simulink model "Trajectory"  (R2025a)
settings: Solver=VariableStepAuto  StartTime=0.0  StopTime=30  FixedStep=0.01  RelTol=1e-3
values from neighbouring files (symbols this model uses):
  P = [     0   0 ... (first row only)    [untitled2.m]
  s = 5    [untitled2.m]
libraries: robotalgslib x1
settings Model: Creator=mwali  LastModifiedBy=mwali

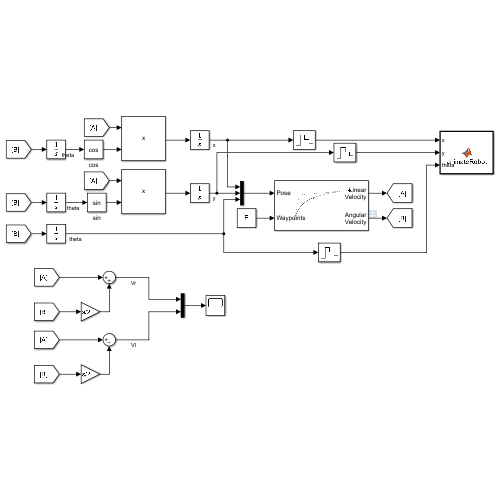
[thumbnail: Simulink's stored preview of the top-level diagram]
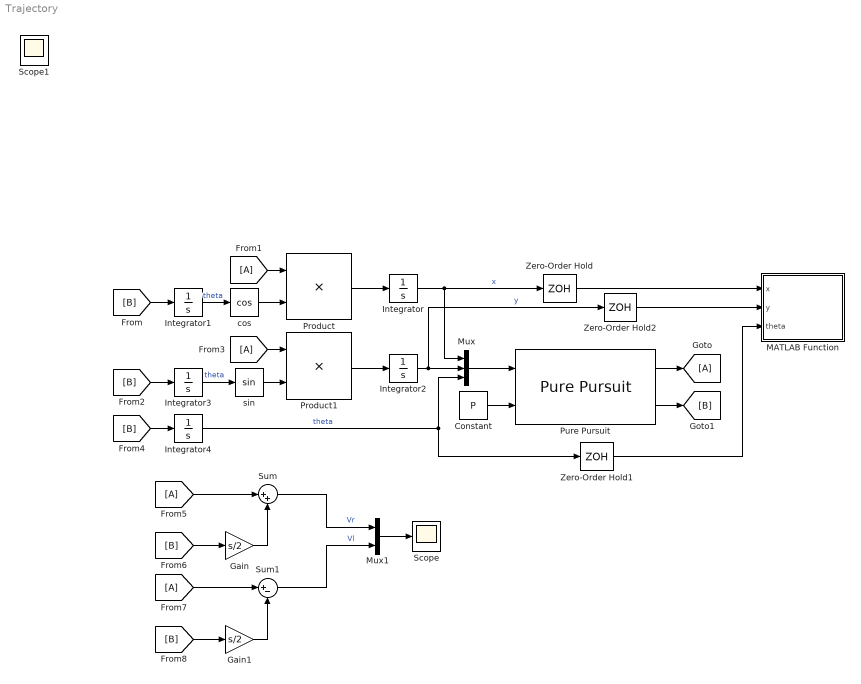
== system Trajectory ==
  Constant : Constant  Value=P
  From{1,3,5,7} (4 alike) : From
  Gain : Gain  Gain=s/2
  Gain1 : Gain  Gain=s/2
  Goto : Goto
  Integrator{,1..4} (5 alike) : Integrator
  MATLAB Function : MATLAB Function  TreatAsAtomicUnit=on
  Mux : Mux  Inputs=3
  Mux1 : Mux  Inputs=2
  Product : Product
  Product1 : Product
  Pure Pursuit : robotalgslib/Pure Pursuit  DesiredLinearVelocityPort=off  DesiredLinearVelocity=0.15  MaxAngularVelocity=1.0  LookaheadDistancePort=off  LookaheadDistance=1.2  TargetDirPort=off  SimulateUsing=Code generation
      settings: LibrarySourceBlock=robotmobilelib/Pure Pursuit
  Scope : Scope
      settings: ActiveDisplayYMinimum=-1.3727035211846959  ActiveDisplayYMaximum=2.3727035211846963
  Sum : Sum  Inputs=|++
  Sum1 : Sum  Inputs=|+-
  Zero-Order Hold : ZeroOrderHold  SampleTime=0.01
  Zero-Order Hold1 : ZeroOrderHold  SampleTime=0.01
  Zero-Order Hold2 : ZeroOrderHold  SampleTime=0.01
  cos : Trigonometry  Operator=cos
  sin : Trigonometry
  Scope1 : Scope
      settings: ActiveDisplayYMinimum=-1  ActiveDisplayYMaximum=1
  wires:
  Product/1 -> Integrator/1
  cos/1 -> Product/2
  Integrator1/1 -> cos/1  "theta"
  [B] -> Integrator1/1
  From1/1 -> Product/1
  Pure Pursuit/1 -> Goto/1
  Pure Pursuit/2 -> [B]
  Integrator/1 -> Zero-Order Hold/1, Mux/1  "x"
  sin/1 -> Product1/2
  Integrator2/1 -> Mux/2, Zero-Order Hold2/1  "y"
  [B] -> Integrator3/1
  Product1/1 -> Integrator2/1
  From3/1 -> Product1/1
  Integrator3/1 -> sin/1  "theta"
  Integrator4/1 -> Zero-Order Hold1/1, Mux/3  "theta"
  [B] -> Integrator4/1
  Mux/1 -> Pure Pursuit/1
  Constant/1 -> Pure Pursuit/2
  Zero-Order Hold/1 -> MATLAB Function/1(x)
  Zero-Order Hold2/1 -> MATLAB Function/2(y)
  Zero-Order Hold1/1 -> MATLAB Function/3(theta)
  [B] -> Gain/1
  From5/1 -> Sum/1
  Gain/1 -> Sum/2
  Sum/1 -> Mux1/1  "Vr"
  From7/1 -> Sum1/1
  Gain1/1 -> Sum1/2
  [B] -> Gain1/1
  Sum1/1 -> Mux1/2  "Vl"
  Mux1/1 -> Scope/1

== matlab function Trajectory/MATLAB Function ==
  data: x input; y input; theta input
function animateRobot(x,y,theta)

persistent hFig hRobot hTrail X Y

% Initialize persistent variables
if isempty(hFig)
    
    hFig = figure('Name','Robot Animation');
    axis equal
    grid on
    hold on
    xlabel('X')
    ylabel('Y')

    % create robot arrow
    hRobot = quiver(x,y,cos(theta),sin(theta),0.5,'LineWidth',2);

    % create trajectory line
    hTrail = plot(x,y,'b-');

    X = x;
    Y = y;

else
    
    % update trajectory
    X(end+1) = x;
    Y(end+1) = y;

    set(hTrail,'XData',X,'YData',Y)

    % update robot direction
    set(hRobot,'XData',x,'YData',y,'UData',cos(theta),'VData',sin(theta))

    drawnow limitrate

end
